simulink model "slidingSimulation"  (R2017a)
settings: Solver=VariableStepAuto  StartTime=0.0  StopTime=tSimul  RelTol=1e-3
values from neighbouring files (symbols this model uses):
  d = 0    [slidingPL.m]    (also in slidingSaturado.m)
  Ldes = 2    [slidingPL.m]    (also in slidingSaturado.m)
  leaderAcceleration = 1    [sliding.m]    (also in slidingPL.m; slidingSaturado.m)
  perf = input('Tipo de lider (perfecto(1), ruidoso(0)):')    [slidingPL.m]    (also in slidingSaturado.m)
  ts = 0.1    [slidingPL.m]    (also in slidingSaturado.m)
  v0Bici1 = 1    [slidingPL.m]    (also in slidingSaturado.m)
  v0Bici2 = 1    [slidingPL.m]    (also in slidingSaturado.m)
  v0Bici3 = 1    [slidingPL.m]    (also in slidingSaturado.m)
  v0Leader = input('Velocidad lider (m/s)(2.7,4.16,5)')    [slidingPL.m]    (also in slidingSaturado.m)
  x0Bici1 = -10    [slidingPL.m]    (also in slidingSaturado.m)
  x0Bici2 = -20    [slidingPL.m]    (also in slidingSaturado.m)
  x0Bici3 = -30    [slidingPL.m]    (also in slidingSaturado.m)
  x0Leader = 0    [slidingPL.m]    (also in slidingSaturado.m)
undefined symbols (not defined in the file or in its folder): slidingFunction
settings Model: Creator=tlara  LastModifiedBy=tlara

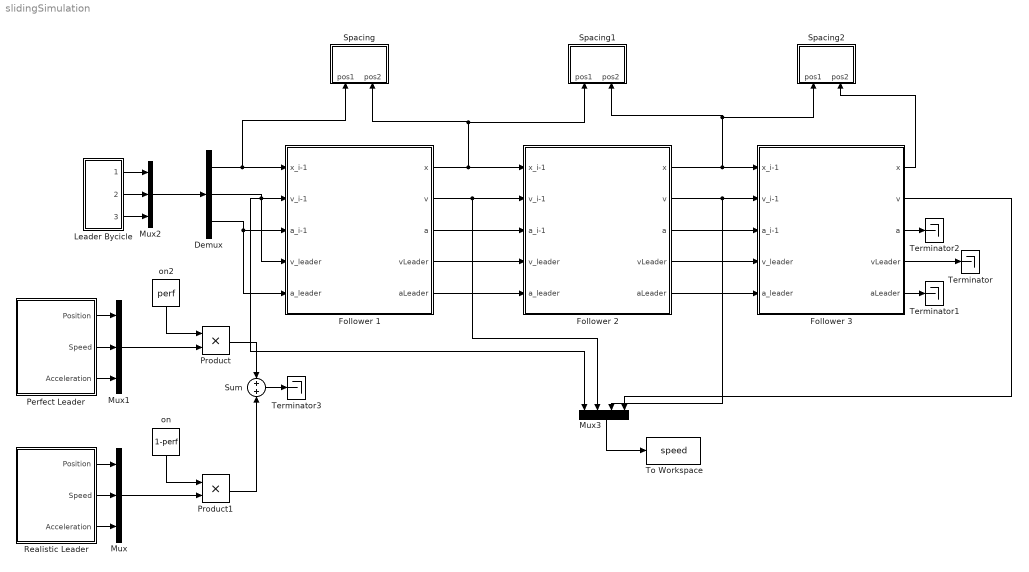
== system slidingSimulation ==
  Demux : Demux  Outputs=3
  "Follower 1 " : Subsystem
  Follower 2 : Subsystem
  "Follower 3 " : Subsystem
  "Leader Bycicle " : Subsystem
  Mux : Mux  Inputs=3
  Mux1 : Mux  Inputs=3
  Mux2 : Mux  Inputs=3
  Mux3 : Mux
  Perfect Leader : Subsystem
  Product : Product
  Product1 : Product
  Realistic Leader : Subsystem
  Spacing : Subsystem
  Spacing1 : Subsystem
  Spacing2 : Subsystem
  Sum : Sum
  Terminator{,1..3} (4 alike) : Terminator
  To Workspace : ToWorkspace  VariableName=speed  SaveFormat=Timeseries  SampleTime=-1
  on : Constant  Value=1-perf
  on2 : Constant  Value=perf
  wires:
  Realistic Leader/1(Position) -> Mux/1
  Realistic Leader/2(Speed) -> Mux/2
  Realistic Leader/3(Acceleration) -> Mux/3
  Perfect Leader/1(Position) -> Mux1/1
  Perfect Leader/2(Speed) -> Mux1/2
  Perfect Leader/3(Acceleration) -> Mux1/3
  Mux1/1 -> Product/2
  Mux/1 -> Product1/2
  on/1 -> Product1/1
  on2/1 -> Product/1
  Product/1 -> Sum/1
  Product1/1 -> Sum/2
  Demux/3 -> "Follower 1 "/5(a_leader), "Follower 1 "/3(a_i-1)
  Demux/2 -> Mux3/1, "Follower 1 "/4(v_leader), "Follower 1 "/2(v_i-1)
  Demux/1 -> Spacing/1(pos1), "Follower 1 "/1("x_i-1 ")
  "Follower 1 "/1(x) -> Spacing1/1(pos1), Spacing/2(pos2), Follower 2/1("x_i-1 ")
  "Follower 1 "/2(v) -> Mux3/2, Follower 2/2(v_i-1)
  "Follower 1 "/3(a) -> Follower 2/3(a_i-1)
  "Follower 1 "/4("vLeader ") -> Follower 2/4(v_leader)
  "Follower 1 "/5(aLeader) -> Follower 2/5(a_leader)
  Follower 2/1(x) -> Spacing2/1(pos1), Spacing1/2(pos2), "Follower 3 "/1("x_i-1 ")
  Follower 2/2(v) -> Mux3/3, "Follower 3 "/2(v_i-1)
  Follower 2/3(a) -> "Follower 3 "/3(a_i-1)
  Follower 2/4("vLeader ") -> "Follower 3 "/4(v_leader)
  Follower 2/5(aLeader) -> "Follower 3 "/5(a_leader)
  "Leader Bycicle "/1(Position) -> Mux2/1
  "Leader Bycicle "/2(Speed) -> Mux2/2
  "Leader Bycicle "/3("Acceleration ") -> Mux2/3
  Mux2/1 -> Demux/1
  "Follower 3 "/1(x) -> Spacing2/2(pos2)
  "Follower 3 "/4("vLeader ") -> Terminator/1
  "Follower 3 "/5(aLeader) -> Terminator1/1
  "Follower 3 "/3(a) -> Terminator2/1
  Mux3/1 -> To Workspace/1
  Sum/1 -> Terminator3/1
  "Follower 3 "/2(v) -> Mux3/4

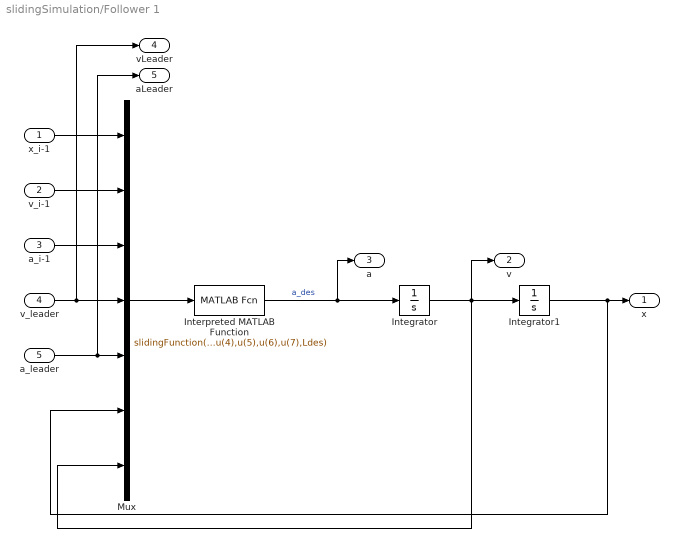
== system slidingSimulation/Follower 1  ==
  "x_i-1 " : Inport
  v_i-1 : Inport  Port=2
  a_i-1 : Inport  Port=3
  v_leader : Inport  Port=4
  a_leader : Inport  Port=5
  Integrator : Integrator  InitialCondition=v0Bici1
  Integrator1 : Integrator  InitialCondition=x0Bici1
  Interpreted MATLAB Function : MATLABFcn  MATLABFcn=slidingFunction(u(1),u(2),u(3),u(4),u(5),u(6),u(7),Ldes)  OutputDimensions=1
  Mux : Mux  Inputs=7
  x : Outport
  v : Outport  Port=2
  a : Outport  Port=3
  "vLeader " : Outport  Port=4
  aLeader : Outport  Port=5
  wires:
  Interpreted MATLAB Function/1 -> a/1, Integrator/1  "a_des"
  Integrator1/1 -> Mux/6, x/1
  Mux/1 -> Interpreted MATLAB Function/1
  Integrator/1 -> Mux/7, v/1, Integrator1/1
  "x_i-1 "/1 -> Mux/1
  v_i-1/1 -> Mux/2
  a_i-1/1 -> Mux/3
  v_leader/1 -> "vLeader "/1, Mux/4
  a_leader/1 -> aLeader/1, Mux/5

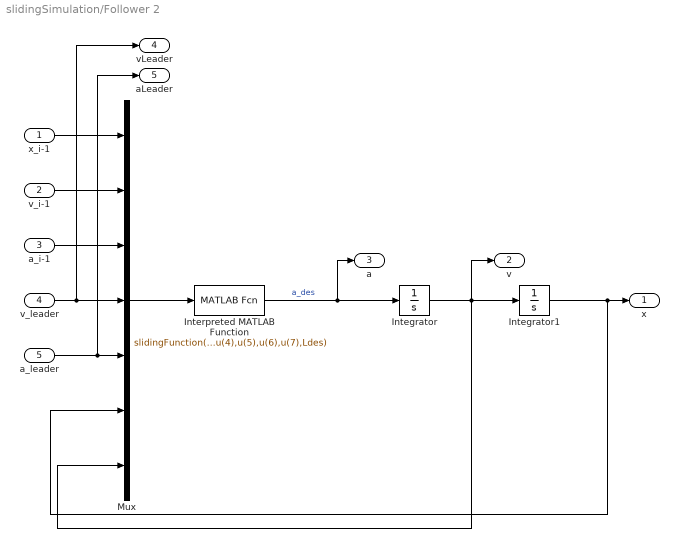
== system slidingSimulation/Follower 2 ==
  "x_i-1 " : Inport
  v_i-1 : Inport  Port=2
  a_i-1 : Inport  Port=3
  v_leader : Inport  Port=4
  a_leader : Inport  Port=5
  Integrator : Integrator  InitialCondition=v0Bici2
  Integrator1 : Integrator  InitialCondition=x0Bici2
  Interpreted MATLAB Function : MATLABFcn  MATLABFcn=slidingFunction(u(1),u(2),u(3),u(4),u(5),u(6),u(7),Ldes)  OutputDimensions=1
  Mux : Mux  Inputs=7
  x : Outport
  v : Outport  Port=2
  a : Outport  Port=3
  "vLeader " : Outport  Port=4
  aLeader : Outport  Port=5
  wires:
  Interpreted MATLAB Function/1 -> a/1, Integrator/1  "a_des"
  Integrator1/1 -> Mux/6, x/1
  Mux/1 -> Interpreted MATLAB Function/1
  Integrator/1 -> Mux/7, v/1, Integrator1/1
  "x_i-1 "/1 -> Mux/1
  v_i-1/1 -> Mux/2
  a_i-1/1 -> Mux/3
  v_leader/1 -> "vLeader "/1, Mux/4
  a_leader/1 -> aLeader/1, Mux/5

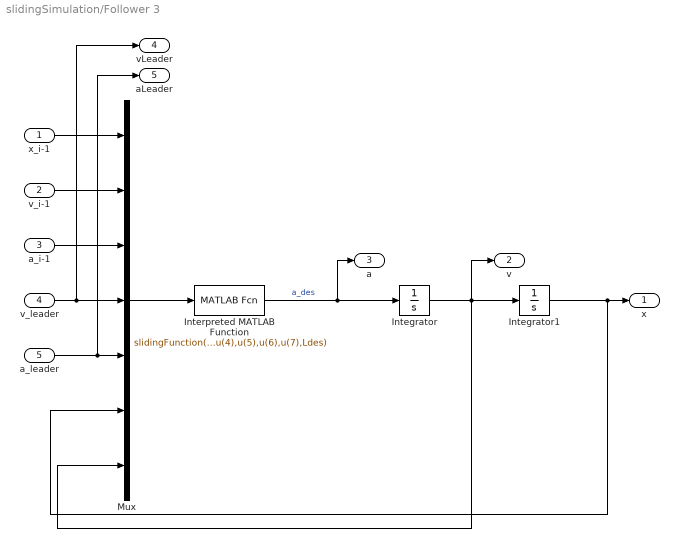
== system slidingSimulation/Follower 3  ==
  "x_i-1 " : Inport
  v_i-1 : Inport  Port=2
  a_i-1 : Inport  Port=3
  v_leader : Inport  Port=4
  a_leader : Inport  Port=5
  Integrator : Integrator  InitialCondition=v0Bici3
  Integrator1 : Integrator  InitialCondition=x0Bici3
  Interpreted MATLAB Function : MATLABFcn  MATLABFcn=slidingFunction(u(1),u(2),u(3),u(4),u(5),u(6),u(7),Ldes)  OutputDimensions=1
  Mux : Mux  Inputs=7
  x : Outport
  v : Outport  Port=2
  a : Outport  Port=3
  "vLeader " : Outport  Port=4
  aLeader : Outport  Port=5
  wires:
  Interpreted MATLAB Function/1 -> a/1, Integrator/1  "a_des"
  Integrator1/1 -> Mux/6, x/1
  Mux/1 -> Interpreted MATLAB Function/1
  Integrator/1 -> Mux/7, v/1, Integrator1/1
  "x_i-1 "/1 -> Mux/1
  v_i-1/1 -> Mux/2
  a_i-1/1 -> Mux/3
  v_leader/1 -> "vLeader "/1, Mux/4
  a_leader/1 -> aLeader/1, Mux/5

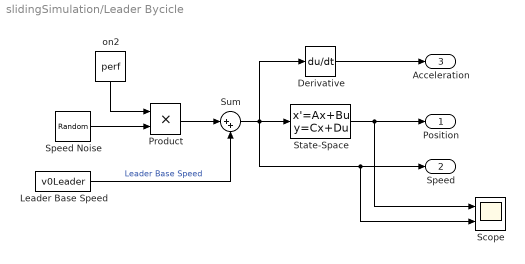
== system slidingSimulation/Leader Bycicle  ==
  Derivative : Derivative
  "Leader Base Speed " : Constant  Value=v0Leader
  Product : Product
  Scope : Scope  NumInputPorts=2
  Speed Noise : RandomNumber  Variance=0.02  SampleTime=ts
  State-Space : StateSpace  A=[0]  B=[1]  C=[1]  D=[0]  X0=[x0Leader]  ContinuousStateAttributes='position'
  Sum : Sum  Inputs=|++
  on2 : Constant  Value=perf
  Position : Outport
  Speed : Outport  Port=2
  "Acceleration " : Outport  Port=3
  wires:
  "Leader Base Speed "/1 -> Sum/2  "Leader Base Speed"
  State-Space/1 -> Position/1, Scope/1
  Sum/1 -> Derivative/1, State-Space/1, Speed/1, Scope/2
  Derivative/1 -> "Acceleration "/1
  Product/1 -> Sum/1
  Speed Noise/1 -> Product/2
  on2/1 -> Product/1

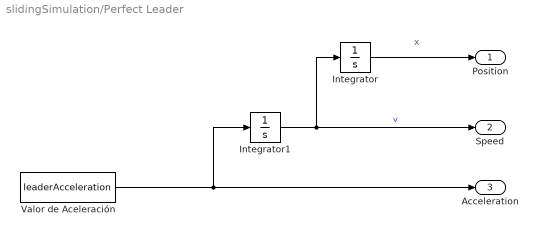
== system slidingSimulation/Perfect Leader ==
  note: x
  Integrator : Integrator
  Integrator1 : Integrator
  Valor de Aceleración : Constant  Value=leaderAcceleration
  Position : Outport
  Speed : Outport  Port=2
  Acceleration : Outport  Port=3
  wires:
  Integrator/1 -> Position/1
  Valor de Aceleración/1 -> Integrator1/1, Acceleration/1
  Integrator1/1 -> Integrator/1, Speed/1  "v"

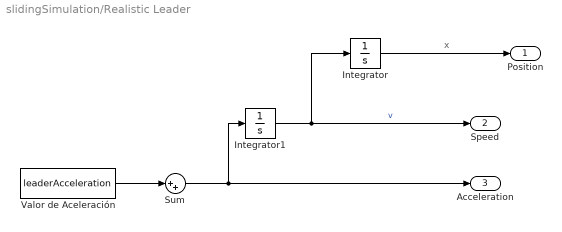
== system slidingSimulation/Realistic Leader ==
  note: x
  Integrator : Integrator
  Integrator1 : Integrator
  Sum : Sum  Inputs=|++
  Valor de Aceleración : Constant  Value=leaderAcceleration
  Position : Outport
  Speed : Outport  Port=2
  Acceleration : Outport  Port=3
  wires:
  Integrator/1 -> Position/1
  Integrator1/1 -> Integrator/1, Speed/1  "v"
  Sum/1 -> Integrator1/1, Acceleration/1
  Valor de Aceleración/1 -> Sum/1

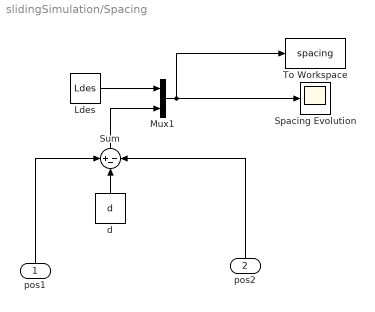
== system slidingSimulation/Spacing ==
  pos1 : Inport
  pos2 : Inport  Port=2
  Ldes : Constant  Value=Ldes
  Mux1 : Mux  Inputs=2
  Spacing Evolution : Scope
  Sum : Sum  Inputs=+--
  To Workspace : ToWorkspace  VariableName=spacing  SaveFormat=Timeseries  SampleTime=-1
  "d " : Constant  Value=d
  wires:
  Ldes/1 -> Mux1/1
  "d "/1 -> Sum/2
  pos2/1 -> Sum/3
  pos1/1 -> Sum/1
  Sum/1 -> Mux1/2
  Mux1/1 -> To Workspace/1, Spacing Evolution/1

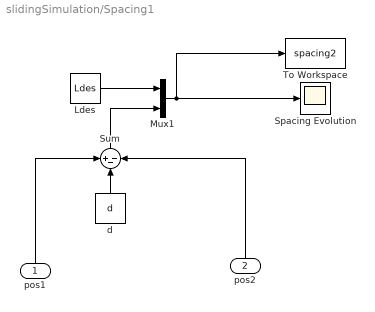
== system slidingSimulation/Spacing1 ==
  pos1 : Inport
  pos2 : Inport  Port=2
  Ldes : Constant  Value=Ldes
  Mux1 : Mux  Inputs=2
  Spacing Evolution : Scope
  Sum : Sum  Inputs=+--
  To Workspace : ToWorkspace  VariableName=spacing2  SaveFormat=Timeseries  SampleTime=-1
  "d " : Constant  Value=d
  wires:
  Ldes/1 -> Mux1/1
  "d "/1 -> Sum/2
  pos2/1 -> Sum/3
  pos1/1 -> Sum/1
  Sum/1 -> Mux1/2
  Mux1/1 -> To Workspace/1, Spacing Evolution/1

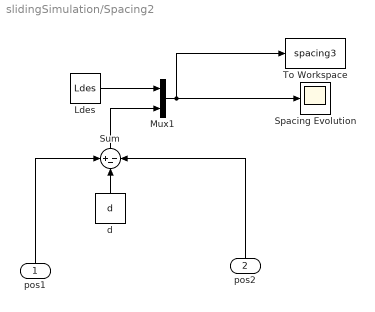
== system slidingSimulation/Spacing2 ==
  pos1 : Inport
  pos2 : Inport  Port=2
  Ldes : Constant  Value=Ldes
  Mux1 : Mux  Inputs=2
  Spacing Evolution : Scope
  Sum : Sum  Inputs=+--
  To Workspace : ToWorkspace  VariableName=spacing3  SaveFormat=Timeseries  SampleTime=-1
  "d " : Constant  Value=d
  wires:
  Ldes/1 -> Mux1/1
  "d "/1 -> Sum/2
  pos2/1 -> Sum/3
  pos1/1 -> Sum/1
  Sum/1 -> Mux1/2
  Mux1/1 -> To Workspace/1, Spacing Evolution/1
